simulink model "sampleModel1446"  (R2023a)
settings: Solver=VariableStepAuto  StartTime=0.0  StopTime=10.0  RelTol=1e-3
libraries: hdlsllib x8, simulink x2
settings Model: Creator=user1  LastModifiedBy=user1

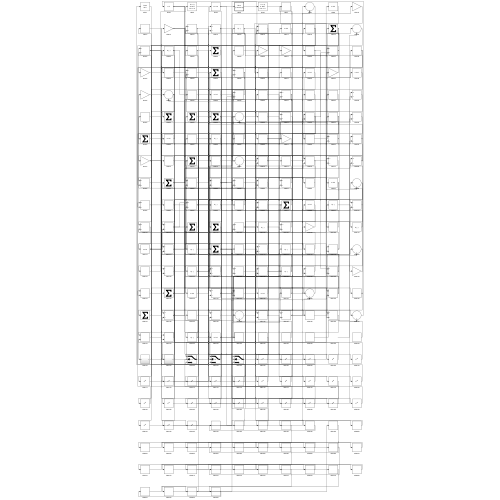
[thumbnail: Simulink's stored preview of the top-level diagram]
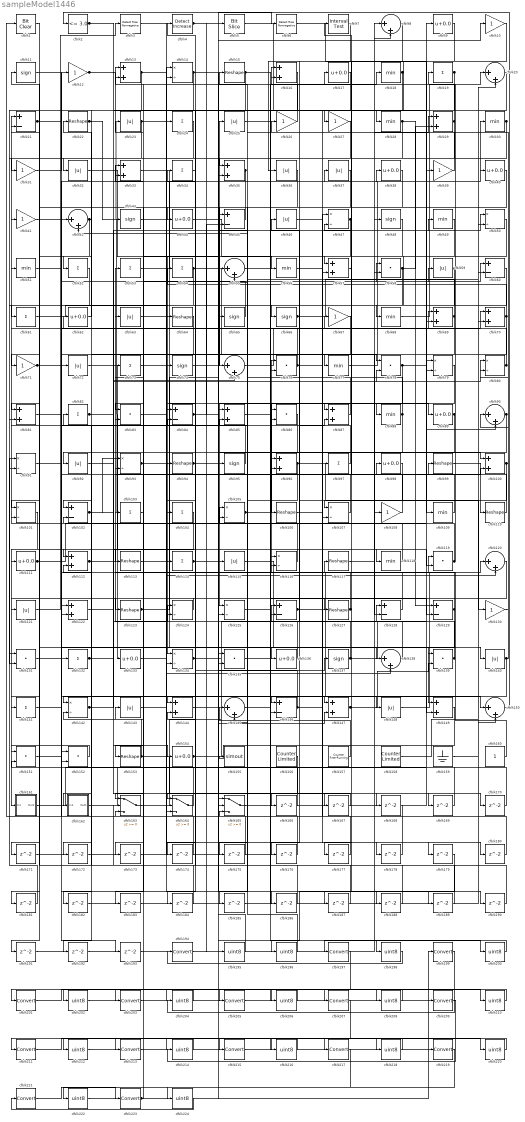
== system sampleModel1446 ==
  cfblk1 : simulink/Logic and Bit Operations/Bit Clear  iBit=0
      settings: LibrarySourceBlock=|
      | hdlsllib/Logic and Bit
      | Operations/Bit Clear
  cfblk{10,12,26..27,31,39,41,67,71,108,130} (11 alike) : Gain
  cfblk{13,16,29,33,35,57,69..70,81,85,87,96,100,112,122,144,147,149} (18 alike) : Sum
  cfblk{14,47,50,79..80,91,93,101,105,107,116,124..125,134,142} (15 alike) : Product  Inputs=*/  RndMeth=Zero  SaturateOnIntegerOverflow=on
  cfblk{21,45,60,84,102,126,128..129,146} (9 alike) : Sum  Inputs=+-
  cfblk{19,24,34,52..54,61,73,82,97,103..104,114,132,141} (15 alike) : Sum  Inputs=+
  cfblk{15,22,64,94,99,106,110,113,117,123,127,153} (12 alike) : Reshape
  cfblk{18,28,30,49,51,56,68,77,88,109,118} (11 alike) : MinMax
  cfblk{11,43,48,65..66,74,95,137} (8 alike) : Signum
  cfblk{9,17,38,40,44,62,89,98,111,133,136,154} (12 alike) : Bias  Bias=0.0  SaturateOnIntegerOverflow=off
  cfblk{23,25,32,36..37,46,59,63,72,92,115,121,140,143,148} (15 alike) : Abs  SaturateOnIntegerOverflow=off
  cfblk{58,76,78,83,86,119,131,135,139,151..152} (11 alike) : DotProduct  OutDataTypeStr=Inherit: Inherit via internal rule
  cfblk{8,20,42,55,75,90,120,138,145,150} (10 alike) : Sum  Inputs=|++
  cfblk155 : ToWorkspace  VariableName=simout  SaveFormat=Timeseries  SampleTime=-1
  cfblk156 : hdlsllib/Sources/Counter Limited  uplimit=7  tsamp=-1
  cfblk157 : hdlsllib/Sources/Counter Free-Running  NumBits=16  tsamp=-1
  cfblk158 : hdlsllib/Sources/Counter Limited  uplimit=7  tsamp=-1
  cfblk159 : Ground
  cfblk160 : Constant  SampleTime=-1
  cfblk161 : Subsystem
      settings: LibrarySourceBlock=|
      | hdlsllib/Ports &
      | Subsystems/Subsystem
  cfblk162 : Subsystem
      settings: LibrarySourceBlock=|
      | hdlsllib/Ports &
      | Subsystems/Subsystem
  cfblk163 : Switch  SaturateOnIntegerOverflow=off  InputSameDT=off
  cfblk164 : Switch  SaturateOnIntegerOverflow=off  InputSameDT=off
  cfblk165 : Switch  SaturateOnIntegerOverflow=off  InputSameDT=off
  cfblk{166..193} (28 alike) : Delay  SampleTime=1
  cfblk{194,197,199,201,203,205,207,209,211,213,215,217,219,221,223} (15 alike) : DataTypeConversion  SaturateOnIntegerOverflow=off  RndMeth=Floor
  cfblk{195..196,198,200,202,204,206,208,210,212,214,216,218,220,222,224} (16 alike) : DataTypeConversion  OutDataTypeStr=uint8  SaturateOnIntegerOverflow=off  RndMeth=Floor
  cfblk2 : hdlsllib/Logic and Bit Operations/Compare To Constant  relop=<=  const=3.0  OutDataTypeStr=boolean
  cfblk3 : hdlsllib/Logic and Bit Operations/Detect Rise Nonnegative  vinit=0  OutDataTypeStr=boolean
  cfblk4 : simulink/Logic and Bit Operations/Detect Increase  vinit=0.0  OutDataTypeStr=boolean
      settings: LibrarySourceBlock=|
      | hdlsllib/Logic and Bit
      | Operations/Detect
      | Increase
  cfblk5 : hdlsllib/Logic and Bit Operations/Bit Slice  lidx=7  ridx=0
  cfblk6 : hdlsllib/Logic and Bit Operations/Detect Rise Nonnegative  vinit=0  OutDataTypeStr=boolean
  cfblk7 : hdlsllib/Logic and Bit Operations/Interval Test  IntervalClosedRight=on  uplimit=0.5  IntervalClosedLeft=on  lowlimit=-0.5  OutDataTypeStr=boolean
  wires:
  cfblk33/1 -> cfblk87/1
  cfblk154/1 -> cfblk128/1, cfblk147/2
  cfblk70/1 -> cfblk92/1, cfblk54/1
  cfblk121/1 -> cfblk3/1
  cfblk12/1 -> cfblk133/1, cfblk114/1, cfblk154/1
  cfblk140/1 -> cfblk26/1, cfblk172/1
  cfblk63/1 -> cfblk136/1
  cfblk47/1 -> cfblk57/1, cfblk65/1
  cfblk118/1 -> cfblk21/1
  cfblk49/1 -> cfblk134/1
  cfblk8/1 -> cfblk36/1
  cfblk44/1 -> cfblk56/1
  cfblk74/1 -> cfblk25/1
  cfblk53/1 -> cfblk38/1
  cfblk19/1 -> cfblk66/1, cfblk61/1
  cfblk68/1 -> cfblk20/1
  cfblk129/1 -> cfblk53/1, cfblk93/2, cfblk191/1
  cfblk115/1 -> cfblk140/1
  cfblk72/1 -> cfblk118/1
  cfblk104/1 -> cfblk161/1(In1)
  cfblk69/1 -> cfblk13/1, cfblk183/1
  cfblk2/1 -> cfblk27/1, cfblk75/2, cfblk135/2
  cfblk48/1 -> cfblk83/1
  cfblk41/1 -> cfblk42/1
  cfblk80/1 -> cfblk74/1, cfblk62/1
  cfblk142/1 -> cfblk87/2, cfblk78/2
  cfblk78/1 -> cfblk125/1, cfblk90/2
  cfblk119/1 -> cfblk105/1, cfblk19/1
  cfblk152/1 -> cfblk151/1
  cfblk15/1 -> cfblk31/1, cfblk129/2
  cfblk82/1 -> cfblk49/1, cfblk80/1
  cfblk133/1 -> cfblk70/1
  cfblk77/1 -> cfblk30/1
  cfblk38/1 -> cfblk75/1
  cfblk136/1 -> cfblk103/1
  cfblk7/1 -> cfblk146/1
  cfblk55/1 -> cfblk40/1
  cfblk60/1 -> cfblk144/1
  cfblk148/1 -> cfblk120/1
  cfblk75/1 -> cfblk8/1
  cfblk105/1 -> cfblk127/1, cfblk170/1
  cfblk151/1 -> cfblk72/1
  cfblk76/1 -> cfblk41/1, cfblk88/1
  cfblk128/1 -> cfblk63/1
  cfblk62/1 -> cfblk22/1
  cfblk117/1 -> cfblk108/1
  cfblk28/1 -> cfblk102/1, cfblk129/1
  cfblk13/1 -> cfblk131/2, cfblk169/1
  cfblk111/1 -> cfblk9/1, cfblk67/1, cfblk100/2
  cfblk127/1 -> cfblk76/1, cfblk76/2
  cfblk10/1 -> cfblk107/1
  cfblk134/1 -> cfblk48/1, cfblk97/1
  cfblk54/1 -> cfblk128/2, cfblk124/2
  cfblk149/1 -> cfblk155/1
  cfblk89/1 -> cfblk153/1, cfblk162/1(In1)
  cfblk4/1 -> cfblk6/1, cfblk195/1
  cfblk102/1 -> cfblk58/1, cfblk93/1
  cfblk164/1 -> cfblk82/1
  cfblk61/1 -> cfblk64/1
  cfblk109/1 -> cfblk47/2
  cfblk5/1 -> cfblk109/1
  cfblk163/1 -> cfblk126/1
  cfblk137/1 -> cfblk79/1, cfblk23/1
  cfblk64/1 -> cfblk142/1
  cfblk156/1 -> cfblk164/1
  cfblk112/1 -> cfblk14/2, cfblk50/1
  cfblk22/1 -> cfblk43/1, cfblk192/1
  cfblk88/1 -> cfblk123/1, cfblk7/1
  cfblk139/1 -> cfblk13/2, cfblk96/2
  cfblk116/1 -> cfblk11/1
  cfblk159/1 -> cfblk70/2
  cfblk93/1 -> cfblk149/1, cfblk138/2
  cfblk113/1 -> cfblk55/1
  cfblk123/1 -> cfblk17/1, cfblk5/1
  cfblk101/1 -> cfblk111/1
  cfblk66/1 -> cfblk8/2, cfblk50/2
  cfblk36/1 -> cfblk95/1
  cfblk162/1(Out1) -> cfblk116/1
  cfblk81/1 -> cfblk37/1
  cfblk14/1 -> cfblk32/1, cfblk148/1
  cfblk122/1 -> cfblk105/2
  cfblk87/1 -> cfblk42/2
  cfblk138/1 -> cfblk45/1
  cfblk145/1 -> cfblk18/1
  cfblk79/1 -> cfblk106/1
  cfblk35/1 -> cfblk113/1, cfblk104/1
  cfblk18/1 -> cfblk146/2, cfblk57/2
  cfblk124/1 -> cfblk121/1
  cfblk94/1 -> cfblk69/1, cfblk184/1
  cfblk71/1 -> cfblk139/1, cfblk149/2
  cfblk40/1 -> cfblk141/1
  cfblk83/1 -> cfblk24/1
  cfblk107/1 -> cfblk33/1
  cfblk91/1 -> cfblk59/1
  cfblk157/1 -> cfblk145/1
  cfblk45/1 -> cfblk44/1
  cfblk42/1 -> cfblk112/1, cfblk81/1
  cfblk56/1 -> cfblk107/2
  cfblk110/1 -> cfblk98/1
  cfblk1/1 -> cfblk101/1
  cfblk158/1 -> cfblk20/2
  cfblk126/1 -> cfblk150/1, cfblk60/2
  cfblk32/1 -> cfblk115/1
  cfblk150/1 -> cfblk2/1
  cfblk100/1 -> cfblk80/2, cfblk166/1
  cfblk141/1 -> cfblk86/1
  cfblk86/1 -> cfblk164/3
  cfblk161/1(Out1) -> cfblk69/2
  cfblk95/1 -> cfblk51/1
  cfblk144/1 -> cfblk137/1
  cfblk65/1 -> cfblk33/2
  cfblk165/1 -> cfblk39/1
  cfblk160/1 -> cfblk119/1
  cfblk24/1 -> cfblk152/2
  cfblk23/1 -> cfblk71/1, cfblk119/2
  cfblk132/1 -> cfblk117/1, cfblk124/1
  cfblk46/1 -> cfblk138/1
  cfblk90/1 -> cfblk94/1, cfblk182/1
  cfblk50/1 -> cfblk68/1
  cfblk73/1 -> cfblk60/1
  cfblk108/1 -> cfblk34/1
  cfblk146/1 -> cfblk4/1, cfblk178/1
  cfblk26/1 -> cfblk16/1
  cfblk6/1 -> cfblk79/2
  cfblk67/1 -> cfblk86/2
  cfblk21/1 -> cfblk132/1, cfblk78/1, cfblk193/1
  cfblk59/1 -> cfblk163/1, cfblk145/2
  cfblk131/1 -> cfblk116/2
  cfblk58/1 -> cfblk91/2, cfblk29/2, cfblk147/1
  cfblk25/1 -> cfblk89/1
  cfblk114/1 -> cfblk125/2, cfblk189/1, cfblk190/1
  cfblk96/1 -> cfblk130/1, cfblk185/1
  cfblk30/1 -> cfblk122/2, cfblk52/1
  cfblk27/1 -> cfblk35/1
  cfblk84/1 -> cfblk100/1, cfblk45/2, cfblk10/1
  cfblk147/1 -> cfblk139/2, cfblk29/1
  cfblk125/1 -> cfblk99/1
  cfblk153/1 -> cfblk165/2, cfblk112/2
  cfblk29/1 -> cfblk16/2, cfblk81/2
  cfblk34/1 -> cfblk84/1
  cfblk99/1 -> cfblk110/1
  cfblk103/1 -> cfblk73/1
  cfblk9/1 -> cfblk28/1
  cfblk31/1 -> cfblk12/1
  cfblk43/1 -> cfblk120/2
  cfblk97/1 -> cfblk46/1
  cfblk130/1 -> cfblk90/1
  cfblk39/1 -> cfblk15/1
  cfblk11/1 -> cfblk77/1
  cfblk166/1 -> cfblk102/2
  cfblk92/1 -> cfblk167/1
  cfblk167/1 -> cfblk164/2
  cfblk106/1 -> cfblk168/1
  cfblk168/1 -> cfblk1/1
  cfblk169/1 -> cfblk144/2
  cfblk170/1 -> cfblk151/2
  cfblk16/1 -> cfblk171/1
  cfblk171/1 -> cfblk14/1
  cfblk172/1 -> cfblk126/2
  cfblk120/1 -> cfblk173/1
  cfblk173/1 -> cfblk134/2
  cfblk20/1 -> cfblk174/1
  cfblk174/1 -> cfblk21/2
  cfblk37/1 -> cfblk175/1
  cfblk175/1 -> cfblk122/1
  cfblk17/1 -> cfblk176/1
  cfblk176/1 -> cfblk83/2
  cfblk57/1 -> cfblk177/1
  cfblk177/1 -> cfblk47/1
  cfblk178/1 -> cfblk131/1
  cfblk143/1 -> cfblk179/1
  cfblk135/1 -> cfblk180/1
  cfblk180/1 -> cfblk152/1
  cfblk52/1 -> cfblk181/1
  cfblk181/1 -> cfblk91/1
  cfblk182/1 -> cfblk150/2
  cfblk183/1 -> cfblk96/1
  cfblk184/1 -> cfblk163/2
  cfblk185/1 -> cfblk165/3
  cfblk51/1 -> cfblk186/1
  cfblk186/1 -> cfblk165/1
  cfblk98/1 -> cfblk187/1
  cfblk187/1 -> cfblk142/2
  cfblk3/1 -> cfblk188/1
  cfblk188/1 -> cfblk101/2
  cfblk189/1 -> cfblk55/2
  cfblk190/1 -> cfblk84/2
  cfblk191/1 -> cfblk35/2
  cfblk192/1 -> cfblk58/2
  cfblk193/1 -> cfblk163/3
  cfblk195/1 -> cfblk85/1
  cfblk179/1 -> cfblk196/1
  cfblk196/1 -> cfblk85/2
  cfblk85/1 -> cfblk198/1
  cfblk198/1 -> cfblk194/1
  cfblk194/1 -> cfblk200/1
  cfblk200/1 -> cfblk197/1
  cfblk197/1 -> cfblk202/1
  cfblk202/1 -> cfblk199/1
  cfblk199/1 -> cfblk204/1
  cfblk204/1 -> cfblk201/1
  cfblk201/1 -> cfblk206/1
  cfblk206/1 -> cfblk203/1
  cfblk203/1 -> cfblk208/1
  cfblk208/1 -> cfblk205/1
  cfblk205/1 -> cfblk210/1
  cfblk210/1 -> cfblk207/1
  cfblk207/1 -> cfblk212/1
  cfblk212/1 -> cfblk209/1
  cfblk209/1 -> cfblk214/1
  cfblk214/1 -> cfblk211/1
  cfblk211/1 -> cfblk216/1
  cfblk216/1 -> cfblk213/1
  cfblk213/1 -> cfblk218/1
  cfblk218/1 -> cfblk215/1
  cfblk215/1 -> cfblk220/1
  cfblk220/1 -> cfblk217/1
  cfblk221/1 -> cfblk223/1
  cfblk217/1 -> cfblk222/1
  cfblk222/1 -> cfblk219/1
  cfblk223/1 -> cfblk135/1, cfblk143/1
  cfblk219/1 -> cfblk224/1
  cfblk224/1 -> cfblk221/1

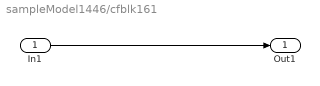
== system sampleModel1446/cfblk161 ==
  In1 : Inport
  Out1 : Outport
  wires:
  In1/1 -> Out1/1

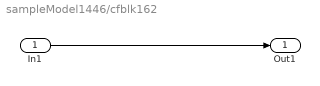
== system sampleModel1446/cfblk162 ==
  In1 : Inport
  Out1 : Outport
  wires:
  In1/1 -> Out1/1
